simulink model "Hierarchical_4Node_Mesh_System"  (R2024b)
settings: Solver=FixedStepAuto  StartTime=0.0  StopTime=210  FixedStep=1  RelTol=1e-3
settings Model: Creator=ARYA MGC  LastModifiedBy=ARYA MGC

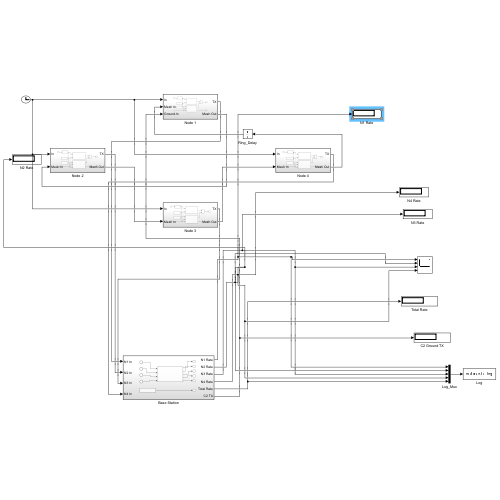
[thumbnail: Simulink's stored preview of the top-level diagram]
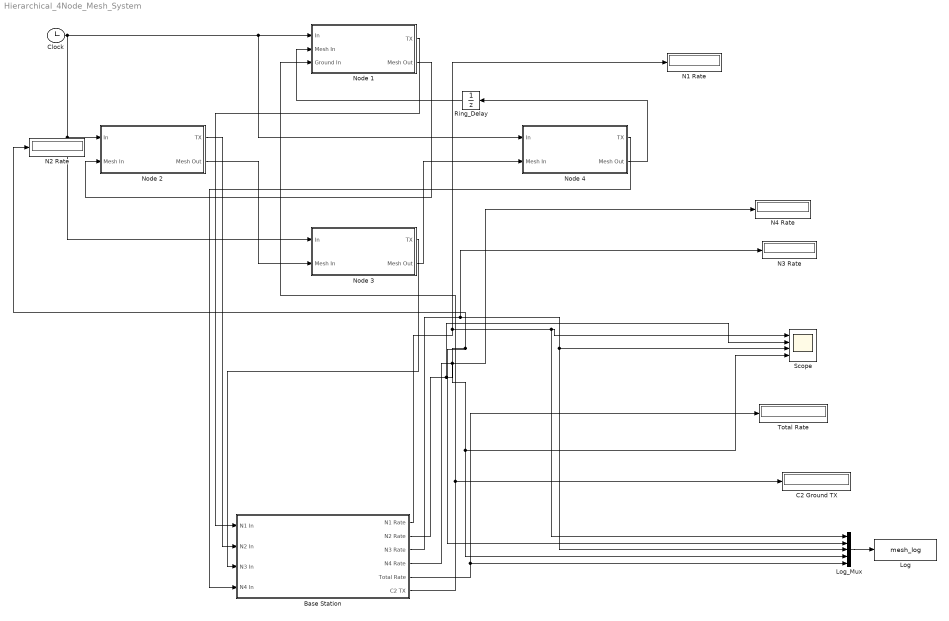
== system Hierarchical_4Node_Mesh_System ==
  Base Station : Subsystem
  C2 Ground TX : Display
  Clock : Clock
  Log : ToWorkspace  VariableName=mesh_log  SampleTime=-1
  Log_Mux : Mux  Inputs=5
  N1 Rate : Display
  N2 Rate : Display
  N3 Rate : Display
  N4 Rate : Display
  Node 1 : Subsystem
  Node 2 : Subsystem
  Node 3 : Subsystem
  Node 4 : Subsystem
  Ring_Delay : UnitDelay  HasFrameUpgradeWarning=on
  Scope : Scope  NumInputPorts=4
  Total Rate : Display
  wires:
  Clock/1 -> Node 1/1(In), Node 4/1(In), Node 2/1(In), Node 3/1(In)
  Node 1/2(Mesh Out) -> Node 2/2(Mesh In)
  Node 2/2(Mesh Out) -> Node 3/2(Mesh In)
  Node 3/2(Mesh Out) -> Node 4/2(Mesh In)
  Node 4/2(Mesh Out) -> Ring_Delay/1
  Ring_Delay/1 -> Node 1/2(Mesh In)
  Node 1/1(TX) -> Base Station/1(N1 In)
  Node 2/1(TX) -> Base Station/2(N2 In)
  Node 3/1(TX) -> Base Station/3(N3 In)
  Node 4/1(TX) -> Base Station/4(N4 In)
  Base Station/1(N1 Rate) -> Scope/1, Log_Mux/1, N1 Rate/1
  Base Station/2(N2 Rate) -> N2 Rate/1, Log_Mux/2, Scope/2
  Base Station/3(N3 Rate) -> Log_Mux/3, Scope/3, N3 Rate/1
  Base Station/4(N4 Rate) -> Scope/4, Log_Mux/4, N4 Rate/1
  Base Station/6(C2 TX) -> Node 1/3(Ground In), C2 Ground TX/1
  Base Station/5(Total Rate) -> Total Rate/1, Log_Mux/5
  Log_Mux/1 -> Log/1

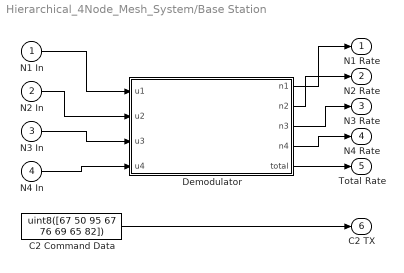
== system Hierarchical_4Node_Mesh_System/Base Station ==
  N1 In : Inport
  N2 In : Inport  Port=2
  N3 In : Inport  Port=3
  N4 In : Inport  Port=4
  C2 Command Data : Constant  Value=uint8([67 50 95 67 76 69 65 82])
  Demodulator : MATLAB Function  TreatAsAtomicUnit=on
  N1 Rate : Outport
  N2 Rate : Outport  Port=2
  N3 Rate : Outport  Port=3
  N4 Rate : Outport  Port=4
  Total Rate : Outport  Port=5
  C2 TX : Outport  Port=6
  wires:
  N1 In/1 -> Demodulator/1(u1)
  N2 In/1 -> Demodulator/2(u2)
  N3 In/1 -> Demodulator/3(u3)
  N4 In/1 -> Demodulator/4(u4)
  Demodulator/1(n1) -> N1 Rate/1
  Demodulator/2(n2) -> N2 Rate/1
  Demodulator/3(n3) -> N3 Rate/1
  Demodulator/4(n4) -> N4 Rate/1
  Demodulator/5(total) -> Total Rate/1
  C2 Command Data/1 -> C2 TX/1

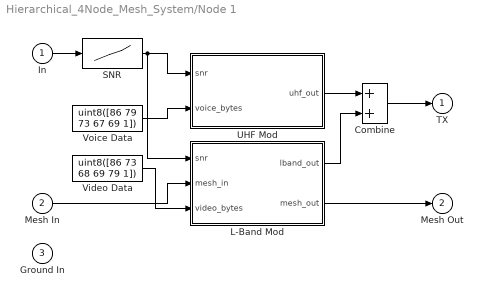
== system Hierarchical_4Node_Mesh_System/Node 1 ==
  In : Inport
  Mesh In : Inport  Port=2
  Ground In : Inport  Port=3
  Combine : Sum
  L-Band Mod : MATLAB Function  TreatAsAtomicUnit=on
  SNR : Lookup_n-D  NumberOfTableDimensions=1  BreakpointsForDimension1=[0 50 51 100 101 160 161 210]  Table=[30 30 18 18 25 25 30 30]  InternalRulePriority=Speed  RndMeth=Simplest
  UHF Mod : MATLAB Function  TreatAsAtomicUnit=on
  Video Data : Constant  Value=uint8([86 73 68 69 79 1])
  Voice Data : Constant  Value=uint8([86 79 73 67 69 1])
  TX : Outport
  Mesh Out : Outport  Port=2
  wires:
  In/1 -> SNR/1
  SNR/1 -> UHF Mod/1(snr), L-Band Mod/1(snr)
  Voice Data/1 -> UHF Mod/2(voice_bytes)
  Mesh In/1 -> L-Band Mod/2(mesh_in)
  Video Data/1 -> L-Band Mod/3(video_bytes)
  UHF Mod/1(uhf_out) -> Combine/1
  L-Band Mod/1(lband_out) -> Combine/2
  Combine/1 -> TX/1
  L-Band Mod/2(mesh_out) -> Mesh Out/1

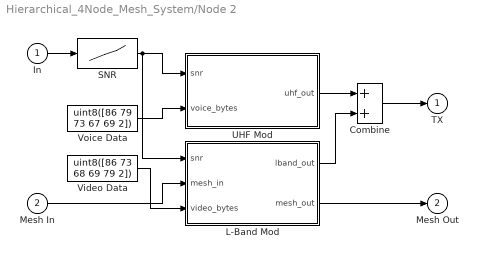
== system Hierarchical_4Node_Mesh_System/Node 2 ==
  In : Inport
  Mesh In : Inport  Port=2
  Combine : Sum
  L-Band Mod : MATLAB Function  TreatAsAtomicUnit=on
  SNR : Lookup_n-D  NumberOfTableDimensions=1  BreakpointsForDimension1=[0 30 31 70 71 110 111 160 161 210]  Table=[22 22 15 15 8 8 12 12 20 20]  InternalRulePriority=Speed  RndMeth=Simplest
  UHF Mod : MATLAB Function  TreatAsAtomicUnit=on
  Video Data : Constant  Value=uint8([86 73 68 69 79 2])
  Voice Data : Constant  Value=uint8([86 79 73 67 69 2])
  TX : Outport
  Mesh Out : Outport  Port=2
  wires:
  In/1 -> SNR/1
  SNR/1 -> UHF Mod/1(snr), L-Band Mod/1(snr)
  Voice Data/1 -> UHF Mod/2(voice_bytes)
  Mesh In/1 -> L-Band Mod/2(mesh_in)
  Video Data/1 -> L-Band Mod/3(video_bytes)
  UHF Mod/1(uhf_out) -> Combine/1
  L-Band Mod/1(lband_out) -> Combine/2
  Combine/1 -> TX/1
  L-Band Mod/2(mesh_out) -> Mesh Out/1

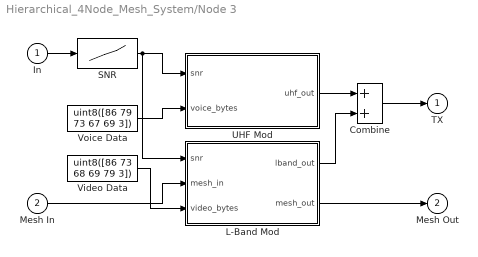
== system Hierarchical_4Node_Mesh_System/Node 3 ==
  In : Inport
  Mesh In : Inport  Port=2
  Combine : Sum
  L-Band Mod : MATLAB Function  TreatAsAtomicUnit=on
  SNR : Lookup_n-D  NumberOfTableDimensions=1  BreakpointsForDimension1=[0 20 21 60 61 120 121 170 171 210]  Table=[20 20 10 10 5 5 8 8 18 18]  InternalRulePriority=Speed  RndMeth=Simplest
  UHF Mod : MATLAB Function  TreatAsAtomicUnit=on
  Video Data : Constant  Value=uint8([86 73 68 69 79 3])
  Voice Data : Constant  Value=uint8([86 79 73 67 69 3])
  TX : Outport
  Mesh Out : Outport  Port=2
  wires:
  In/1 -> SNR/1
  SNR/1 -> UHF Mod/1(snr), L-Band Mod/1(snr)
  Voice Data/1 -> UHF Mod/2(voice_bytes)
  Mesh In/1 -> L-Band Mod/2(mesh_in)
  Video Data/1 -> L-Band Mod/3(video_bytes)
  UHF Mod/1(uhf_out) -> Combine/1
  L-Band Mod/1(lband_out) -> Combine/2
  Combine/1 -> TX/1
  L-Band Mod/2(mesh_out) -> Mesh Out/1

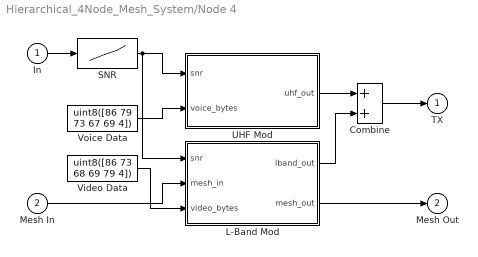
== system Hierarchical_4Node_Mesh_System/Node 4 ==
  In : Inport
  Mesh In : Inport  Port=2
  Combine : Sum
  L-Band Mod : MATLAB Function  TreatAsAtomicUnit=on
  SNR : Lookup_n-D  NumberOfTableDimensions=1  BreakpointsForDimension1=[0 50 51 150 151 210]  Table=[25 25 20 20 25 25]  InternalRulePriority=Speed  RndMeth=Simplest
  UHF Mod : MATLAB Function  TreatAsAtomicUnit=on
  Video Data : Constant  Value=uint8([86 73 68 69 79 4])
  Voice Data : Constant  Value=uint8([86 79 73 67 69 4])
  TX : Outport
  Mesh Out : Outport  Port=2
  wires:
  In/1 -> SNR/1
  SNR/1 -> UHF Mod/1(snr), L-Band Mod/1(snr)
  Voice Data/1 -> UHF Mod/2(voice_bytes)
  Mesh In/1 -> L-Band Mod/2(mesh_in)
  Video Data/1 -> L-Band Mod/3(video_bytes)
  UHF Mod/1(uhf_out) -> Combine/1
  L-Band Mod/1(lband_out) -> Combine/2
  Combine/1 -> TX/1
  L-Band Mod/2(mesh_out) -> Mesh Out/1

== matlab function Hierarchical_4Node_Mesh_System/Node 1/L-Band Mod ==
  data: snr input; lband_out output; mesh_in input; video_bytes input; mesh_out output
function [lband_out, mesh_out] = fcn(snr, mesh_in, video_bytes)
%% L-BAND ADAPTIVE MODULATOR (1.55-1.65 GHz Video Channel)
coder.extrinsic('process_lband_tx_sub');
lband_out = double(0); mesh_out = double(0);
[lband_out, mesh_out] = process_lband_tx_sub(snr, mesh_in, video_bytes);

== matlab function Hierarchical_4Node_Mesh_System/Node 1/UHF Mod ==
  data: snr input; uhf_out output; voice_bytes input
function uhf_out = fcn(snr, voice_bytes)
%% UHF ADAPTIVE MODULATOR (380-400 MHz Voice Channel)
coder.extrinsic('process_uhf_tx_sub');
uhf_out = double(0);
uhf_out = process_uhf_tx_sub(snr, voice_bytes);

== matlab function Hierarchical_4Node_Mesh_System/Node 2/UHF Mod ==
  data: snr input; uhf_out output; voice_bytes input
function uhf_out = fcn(snr, voice_bytes)
%% UHF ADAPTIVE MODULATOR (380-400 MHz Voice Channel)
coder.extrinsic('process_uhf_tx_sub');
uhf_out = double(0);
uhf_out = process_uhf_tx_sub(snr, voice_bytes);

== matlab function Hierarchical_4Node_Mesh_System/Node 2/L-Band Mod ==
  data: snr input; lband_out output; mesh_in input; video_bytes input; mesh_out output
function [lband_out, mesh_out] = fcn(snr, mesh_in, video_bytes)
%% L-BAND ADAPTIVE MODULATOR (1.55-1.65 GHz Video Channel)
coder.extrinsic('process_lband_tx_sub');
lband_out = double(0); mesh_out = double(0);
[lband_out, mesh_out] = process_lband_tx_sub(snr, mesh_in, video_bytes);

== matlab function Hierarchical_4Node_Mesh_System/Node 3/UHF Mod ==
  data: snr input; uhf_out output; voice_bytes input
function uhf_out = fcn(snr, voice_bytes)
%% UHF ADAPTIVE MODULATOR (380-400 MHz Voice Channel)
coder.extrinsic('process_uhf_tx_sub');
uhf_out = double(0);
uhf_out = process_uhf_tx_sub(snr, voice_bytes);

== matlab function Hierarchical_4Node_Mesh_System/Node 3/L-Band Mod ==
  data: snr input; lband_out output; mesh_in input; video_bytes input; mesh_out output
function [lband_out, mesh_out] = fcn(snr, mesh_in, video_bytes)
%% L-BAND ADAPTIVE MODULATOR (1.55-1.65 GHz Video Channel)
coder.extrinsic('process_lband_tx_sub');
lband_out = double(0); mesh_out = double(0);
[lband_out, mesh_out] = process_lband_tx_sub(snr, mesh_in, video_bytes);

== matlab function Hierarchical_4Node_Mesh_System/Node 4/UHF Mod ==
  data: snr input; uhf_out output; voice_bytes input
function uhf_out = fcn(snr, voice_bytes)
%% UHF ADAPTIVE MODULATOR (380-400 MHz Voice Channel)
coder.extrinsic('process_uhf_tx_sub');
uhf_out = double(0);
uhf_out = process_uhf_tx_sub(snr, voice_bytes);

== matlab function Hierarchical_4Node_Mesh_System/Node 4/L-Band Mod ==
  data: snr input; lband_out output; mesh_in input; video_bytes input; mesh_out output
function [lband_out, mesh_out] = fcn(snr, mesh_in, video_bytes)
%% L-BAND ADAPTIVE MODULATOR (1.55-1.65 GHz Video Channel)
coder.extrinsic('process_lband_tx_sub');
lband_out = double(0); mesh_out = double(0);
[lband_out, mesh_out] = process_lband_tx_sub(snr, mesh_in, video_bytes);

== matlab function Hierarchical_4Node_Mesh_System/Base Station/Demodulator ==
  data: u1 input; n1 output; u2 input; u3 input; u4 input; n2 output; n3 output; n4 output; total output
function [n1, n2, n3, n4, total] = fcn(u1, u2, u3, u4)
%% BASE STATION DEMODULATOR
n1 = double(u1); n2 = double(u2); n3 = double(u3); n4 = double(u4);
total = n1 + n2 + n3 + n4;
